simulink model "FYP_Flywheel_Integrated_20260921_182601"  (R2024a)
settings: Solver=FixedStepDiscrete  StartTime=0  StopTime=90  FixedStep=5.0000000000000002e-05  RelTol=1e-3
PostLoadFcn:
  | addpath(fileparts(get_param(bdroot,'FileName')));
model workspace (MAT data in the model file):
  fyp_case.name = '06_combined_dispatch'
  fyp_case.profile = [0 0.0342672001308 0.0685344002617 0.102801600393 0.137068800523 0.171336000654 0.205603200785 0.239870400916 0.274137601047 0.308404801178 0.342672001308 0.376939201439 ... (3010 elements, 602x5)]
  fyp_case.on = 1
  fyp_case.block = 0
  fyp_case.stiff = 0
  fyp_case.fixture = 0
  fyp_case.pwm = 0
  fyp_case.task = 20
  fyp_case.restore = 70
  fyp_case.n0 = 3000
  fyp_case.V0 = 57
  fyp_case.substeps = 1
  fyp_case.speed_pi = 1
  fyp_case.variant = 2
  fyp_controller.R = 0.8
  fyp_controller.L = 0.02
  fyp_controller.Ke = 0.05
  fyp_controller.Kt = 0.05
  fyp_controller.J = 0.51
  fyp_controller.b = 0.001
  fyp_controller.Tc = 0.05
  fyp_controller.Ron = 0.02
  fyp_controller.Rd = 0.01
  fyp_controller.Vf = 0.7
  fyp_controller.td = 1e-06
  fyp_controller.ton = 5e-08
  fyp_controller.toff = 5e-08
  fyp_controller.Ceq = 6e-10
  fyp_controller.Qg = 3e-08
  fyp_controller.Vg = 10
  fyp_controller.blend = 0.5
  fyp_controller.Vs = 60
  fyp_controller.Rs = 0.3
  fyp_controller.C = 0.1
  fyp_controller.fsw = 20000
  fyp_controller.outer = 0.01
  fyp_controller.Imax = 20
  fyp_controller.nmin = 2850
  fyp_controller.nmax = 3150
  fyp_controller.soft = 20
  fyp_controller.hyst = 5
  fyp_controller.Vcharge = 61
  fyp_controller.Vdischarge = 59.5
  fyp_controller.Kg = 80
  fyp_controller.chop_on = 68
  fyp_controller.chop_band = 2
  fyp_controller.Rchop = 6
  fyp_controller.Kp = 25.1327412287
  fyp_controller.Ki = 1030.44239038
  fyp_controller.restore_gain = 4
  fyp_controller.restore_rpm = 3000
  fyp_controller.credit_decay = 0.02
  fyp_controller.credit_margin = 0.9
  fyp_controller.credit_reserve = 5
  fyp_controller.credit_time = 0.2
  fyp_controller.loss_fraction = 0.25
  fyp_controller.speed_Kp = 10.18
  fyp_controller.speed_Ki = 2.55
  fyp_plant.R = 1
  fyp_plant.L = 0.014
  fyp_plant.Ke = 0.05
  fyp_plant.Kt = 0.05
  fyp_plant.J = 0.65
  fyp_plant.b = 0.0015
  fyp_plant.Tc = 0.075
  fyp_plant.Ron = 0.03
  fyp_plant.Rd = 0.015
  fyp_plant.Vf = 0.8
  fyp_plant.td = 2e-06
  fyp_plant.ton = 5e-08
  fyp_plant.toff = 5e-08
  fyp_plant.Ceq = 6e-10
  fyp_plant.Qg = 3e-08
  fyp_plant.Vg = 10
  fyp_plant.blend = 0.5
  fyp_plant.Vs = 57
  fyp_plant.Rs = 0.45
  fyp_plant.C = 0.08
  fyp_plant.fsw = 20000
  fyp_plant.outer = 0.01
  fyp_plant.Imax = 20
  fyp_plant.nmin = 2850
  fyp_plant.nmax = 3150
  fyp_plant.soft = 20
  fyp_plant.hyst = 5
  fyp_plant.Vcharge = 61
  fyp_plant.Vdischarge = 59.5
  fyp_plant.Kg = 80
  fyp_plant.chop_on = 68
  fyp_plant.chop_band = 2
  fyp_plant.Rchop = 6
  fyp_plant.Kp = 25.1327412287
  fyp_plant.Ki = 1030.44239038
  fyp_plant.restore_gain = 4
  fyp_plant.restore_rpm = 3000
  fyp_plant.credit_decay = 0.02
  fyp_plant.credit_margin = 0.9
  fyp_plant.credit_reserve = 5
  fyp_plant.credit_time = 0.2
  fyp_plant.loss_fraction = 0.25
  fyp_plant.speed_Kp = 10.18
  fyp_plant.speed_Ki = 2.55
settings Model: Creator=cheng  LastModifiedBy=cheng
settings DataIOCC: SaveOutput=off  SignalLogging=off  SaveTime=off

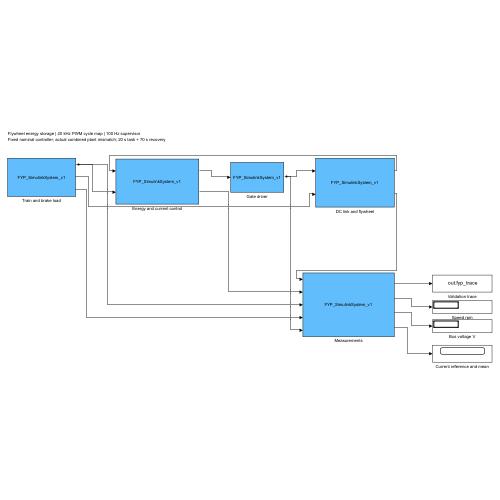
[thumbnail: Simulink's stored preview of the top-level diagram]
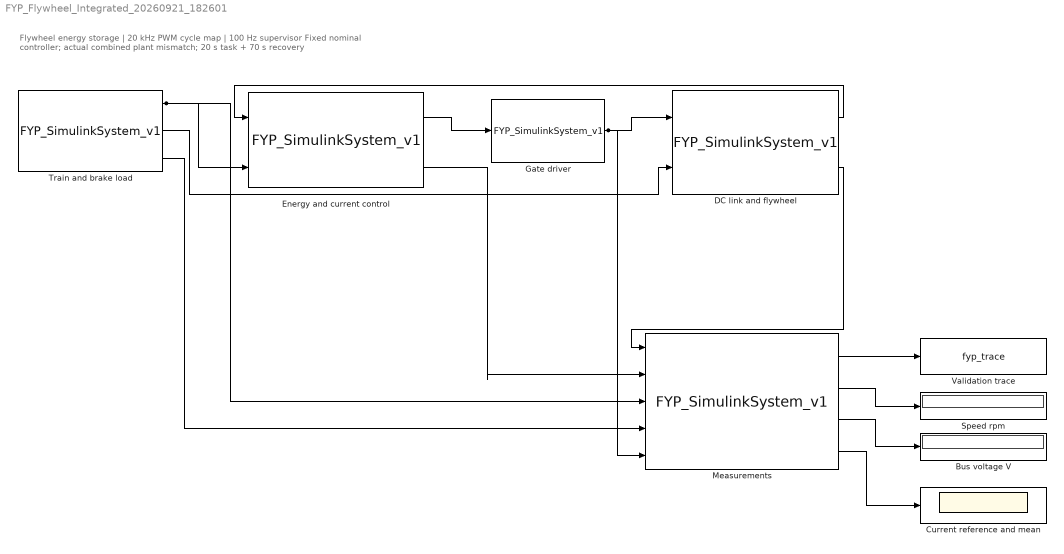
== system FYP_Flywheel_Integrated_20260921_182601 ==
  note: Flywheel energy storage | 20 kHz PWM cycle map | 100 Hz supervisor
      | Fixed nominal controller; actual combined plant mismatch; 20 s task + 70 s recovery
  Bus voltage V : Display
  Current reference and mean : Scope
  DC link and flywheel : M-S-Function  FunctionName=FYP_SimulinkSystem_v1  Parameters='plant',fyp_plant,fyp_case
  Energy and current control : M-S-Function  FunctionName=FYP_SimulinkSystem_v1  Parameters='controller',fyp_controller,fyp_case
  Gate driver : M-S-Function  FunctionName=FYP_SimulinkSystem_v1  Parameters='driver',fyp_plant,fyp_case
  Measurements : M-S-Function  FunctionName=FYP_SimulinkSystem_v1  Parameters='observer',fyp_plant,fyp_case
  Speed rpm : Display
  Train and brake load : M-S-Function  FunctionName=FYP_SimulinkSystem_v1  Parameters='load',fyp_controller,fyp_case
  Validation trace : ToWorkspace  VariableName=fyp_trace  SaveFormat=Structure With Time  SampleTime=-1
      settings: Decimation=200
  wires:
  Train and brake load/1 -> Energy and current control/2, Measurements/3
  Energy and current control/1 -> Gate driver/1
  Gate driver/1 -> DC link and flywheel/1, Measurements/5
  Train and brake load/2 -> DC link and flywheel/2
  DC link and flywheel/1 -> Energy and current control/1
  DC link and flywheel/2 -> Measurements/1
  Energy and current control/2 -> Measurements/2
  Train and brake load/3 -> Measurements/4
  Measurements/1 -> Validation trace/1
  Measurements/2 -> Speed rpm/1
  Measurements/3 -> Bus voltage V/1
  Measurements/4 -> Current reference and mean/1
